simulink model "PIDController"  (R2019a)
settings: Solver=ode5  StartTime=0.0  StopTime=inf  FixedStep=0.01  RelTol=1e-3
settings Model: Creator=Admin  LastModifiedBy=Admin
settings DataIOCC: ReturnWorkspaceOutputs=off
settings DebuggingCC: ArithmeticOperatorsInVariantConditions=warning
settings SFSimCC: SimUseLocalCustomCode=off
settings RTWCC: RTWUseLocalCustomCode=off
settings CodeAppCC: StateflowObjectComments=on

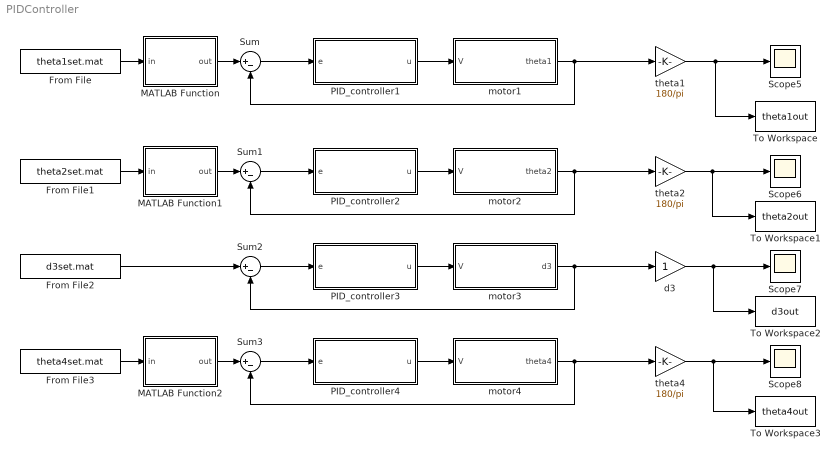
== system PIDController ==
  From File : FromFile  FileName=theta1set.mat
  From File1 : FromFile  FileName=theta2set.mat
  From File2 : FromFile  FileName=d3set.mat
  From File3 : FromFile  FileName=theta4set.mat
  MATLAB Function : MATLAB Function  TreatAsAtomicUnit=on
  MATLAB Function1 : MATLAB Function  TreatAsAtomicUnit=on
  MATLAB Function2 : MATLAB Function  TreatAsAtomicUnit=on
  PID_controller1 : Subsystem  mask{Kp=500, Ki=0, Kd=0}
  PID_controller2 : Subsystem  mask{Kp=500, Ki=0, Kd=0}
  PID_controller3 : Subsystem  mask{Kp=500, Ki=0, Kd=0}
  PID_controller4 : Subsystem  mask{Kp=500, Ki=0, Kd=0}
  Scope{5..8} (4 alike) : Scope
  Sum{,1..3} (4 alike) : Sum  Inputs=|+-
  To Workspace : ToWorkspace  VariableName=theta1out  SampleTime=-1
  To Workspace1 : ToWorkspace  VariableName=theta2out  SampleTime=-1
  To Workspace2 : ToWorkspace  VariableName=d3out  SampleTime=-1
  To Workspace3 : ToWorkspace  VariableName=theta4out  SampleTime=-1
  d3 : Gain
  motor1 : Subsystem  mask{Ki=0.1, Kb=0.1, L=0.5, R=2, Jeff=0.02, Beff=0.2, N=100}
  motor2 : Subsystem  mask{Ki=0.1, Kb=0.1, L=0.5, R=2, Jeff=0.02, Beff=0.2, N=100}
  motor3 : Subsystem  mask{Ki=0.1, Kb=0.1, L=0.5, R=2, Jeff=0.02, Beff=0.2, N=100}
  motor4 : Subsystem  mask{Ki=0.1, Kb=0.1, L=0.5, R=2, Jeff=0.02, Beff=0.2, N=100}
  theta1 : Gain  Gain=180/pi
  theta2 : Gain  Gain=180/pi
  theta4 : Gain  Gain=180/pi
  wires:
  Sum/1 -> PID_controller1/1(e)
  PID_controller1/1(u) -> motor1/1(V)
  Sum1/1 -> PID_controller2/1(e)
  PID_controller2/1(u) -> motor2/1(V)
  Sum2/1 -> PID_controller3/1(e)
  PID_controller3/1(u) -> motor3/1(V)
  Sum3/1 -> PID_controller4/1(e)
  PID_controller4/1(u) -> motor4/1(V)
  From File2/1 -> Sum2/1
  theta4/1 -> To Workspace3/1, Scope8/1
  theta1/1 -> To Workspace/1, Scope5/1
  theta2/1 -> To Workspace1/1, Scope6/1
  motor3/1(d3) -> d3/1, Sum2/2
  d3/1 -> To Workspace2/1, Scope7/1
  From File/1 -> MATLAB Function/1(in)
  From File1/1 -> MATLAB Function1/1(in)
  From File3/1 -> MATLAB Function2/1(in)
  motor4/1(theta4) -> theta4/1, Sum3/2
  motor2/1(theta2) -> theta2/1, Sum1/2
  motor1/1(theta1) -> theta1/1, Sum/2
  MATLAB Function/1(out) -> Sum/1
  MATLAB Function1/1(out) -> Sum1/1
  MATLAB Function2/1(out) -> Sum3/1

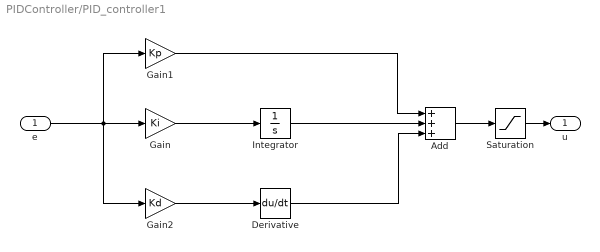
== system PIDController/PID_controller1 ==
  e : Inport
  Add : Sum  Inputs=+++
  Derivative : Derivative
  Gain : Gain  Gain=Ki
  Gain1 : Gain  Gain=Kp
  Gain2 : Gain  Gain=Kd
  Integrator : Integrator
  Saturation : Saturate  UpperLimit=300  LowerLimit=-300
  u : Outport
  wires:
  e/1 -> Gain2/1, Gain1/1, Gain/1
  Gain/1 -> Integrator/1
  Gain2/1 -> Derivative/1
  Gain1/1 -> Add/1
  Integrator/1 -> Add/2
  Derivative/1 -> Add/3
  Add/1 -> Saturation/1
  Saturation/1 -> u/1

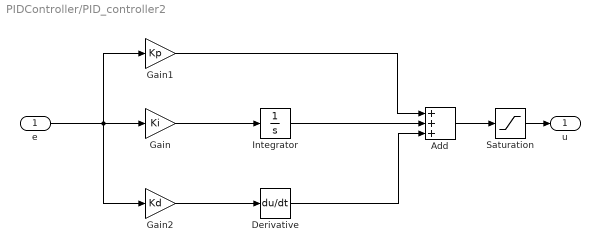
== system PIDController/PID_controller2 ==
  e : Inport
  Add : Sum  Inputs=+++
  Derivative : Derivative
  Gain : Gain  Gain=Ki
  Gain1 : Gain  Gain=Kp
  Gain2 : Gain  Gain=Kd
  Integrator : Integrator
  Saturation : Saturate  UpperLimit=300  LowerLimit=-300
  u : Outport
  wires:
  e/1 -> Gain2/1, Gain1/1, Gain/1
  Gain/1 -> Integrator/1
  Gain2/1 -> Derivative/1
  Gain1/1 -> Add/1
  Integrator/1 -> Add/2
  Derivative/1 -> Add/3
  Add/1 -> Saturation/1
  Saturation/1 -> u/1

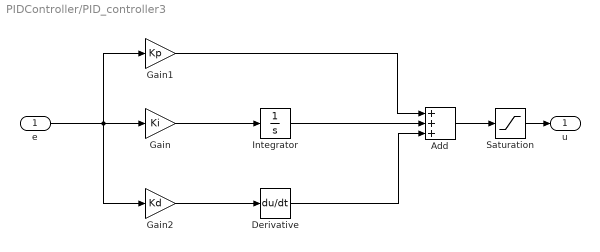
== system PIDController/PID_controller3 ==
  e : Inport
  Add : Sum  Inputs=+++
  Derivative : Derivative
  Gain : Gain  Gain=Ki
  Gain1 : Gain  Gain=Kp
  Gain2 : Gain  Gain=Kd
  Integrator : Integrator
  Saturation : Saturate  UpperLimit=300  LowerLimit=-300
  u : Outport
  wires:
  e/1 -> Gain2/1, Gain1/1, Gain/1
  Gain/1 -> Integrator/1
  Gain2/1 -> Derivative/1
  Gain1/1 -> Add/1
  Integrator/1 -> Add/2
  Derivative/1 -> Add/3
  Add/1 -> Saturation/1
  Saturation/1 -> u/1

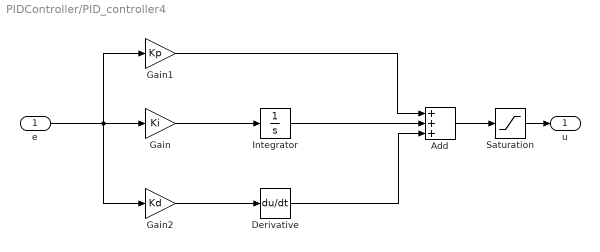
== system PIDController/PID_controller4 ==
  e : Inport
  Add : Sum  Inputs=+++
  Derivative : Derivative
  Gain : Gain  Gain=Ki
  Gain1 : Gain  Gain=Kp
  Gain2 : Gain  Gain=Kd
  Integrator : Integrator
  Saturation : Saturate  UpperLimit=300  LowerLimit=-300
  u : Outport
  wires:
  e/1 -> Gain2/1, Gain1/1, Gain/1
  Gain/1 -> Integrator/1
  Gain2/1 -> Derivative/1
  Gain1/1 -> Add/1
  Integrator/1 -> Add/2
  Derivative/1 -> Add/3
  Add/1 -> Saturation/1
  Saturation/1 -> u/1

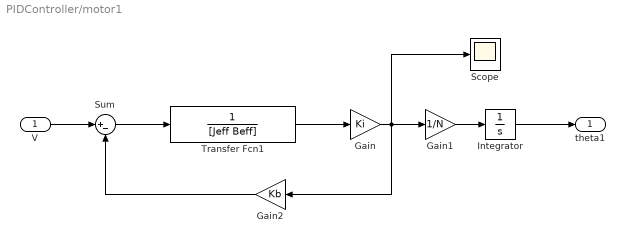
== system PIDController/motor1 ==
  V : Inport
  Gain : Gain  Gain=Ki
  Gain1 : Gain  Gain=1/N
  Gain2 : Gain  Gain=Kb
  Integrator : Integrator
  Scope : Scope
  Sum : Sum  Inputs=|+-
  Transfer Fcn1 : TransferFcn  Denominator=[Jeff Beff]
  theta1 : Outport
  wires:
  Transfer Fcn1/1 -> Gain/1
  Gain2/1 -> Sum/2
  V/1 -> Sum/1
  Sum/1 -> Transfer Fcn1/1
  Gain/1 -> Gain1/1, Gain2/1, Scope/1
  Gain1/1 -> Integrator/1
  Integrator/1 -> theta1/1

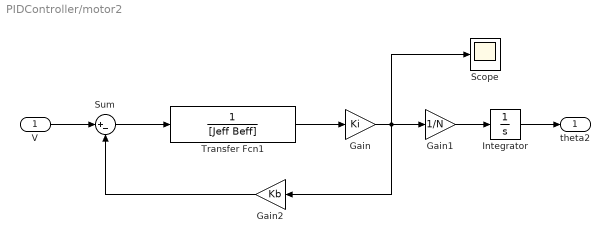
== system PIDController/motor2 ==
  V : Inport
  Gain : Gain  Gain=Ki
  Gain1 : Gain  Gain=1/N
  Gain2 : Gain  Gain=Kb
  Integrator : Integrator  InitialCondition=1.57
  Scope : Scope
  Sum : Sum  Inputs=|+-
  Transfer Fcn1 : TransferFcn  Denominator=[Jeff Beff]
  theta2 : Outport
  wires:
  Transfer Fcn1/1 -> Gain/1
  Gain1/1 -> Integrator/1
  Gain2/1 -> Sum/2
  V/1 -> Sum/1
  Sum/1 -> Transfer Fcn1/1
  Gain/1 -> Gain1/1, Gain2/1, Scope/1
  Integrator/1 -> theta2/1

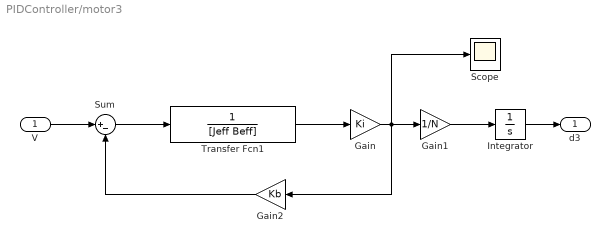
== system PIDController/motor3 ==
  V : Inport
  Gain : Gain  Gain=Ki
  Gain1 : Gain  Gain=1/N
  Gain2 : Gain  Gain=Kb
  Integrator : Integrator
  Scope : Scope
  Sum : Sum  Inputs=|+-
  Transfer Fcn1 : TransferFcn  Denominator=[Jeff Beff]
  d3 : Outport
  wires:
  Transfer Fcn1/1 -> Gain/1
  Gain1/1 -> Integrator/1
  Integrator/1 -> d3/1
  Gain2/1 -> Sum/2
  V/1 -> Sum/1
  Sum/1 -> Transfer Fcn1/1
  Gain/1 -> Gain1/1, Gain2/1, Scope/1

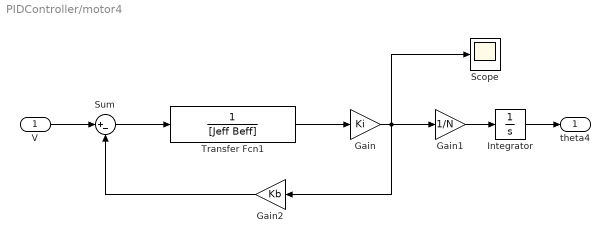
== system PIDController/motor4 ==
  V : Inport
  Gain : Gain  Gain=Ki
  Gain1 : Gain  Gain=1/N
  Gain2 : Gain  Gain=Kb
  Integrator : Integrator  InitialCondition=-1.57
  Scope : Scope
  Sum : Sum  Inputs=|+-
  Transfer Fcn1 : TransferFcn  Denominator=[Jeff Beff]
  theta4 : Outport
  wires:
  Transfer Fcn1/1 -> Gain/1
  Gain/1 -> Gain1/1, Gain2/1, Scope/1
  Gain1/1 -> Integrator/1
  Gain2/1 -> Sum/2
  V/1 -> Sum/1
  Sum/1 -> Transfer Fcn1/1
  Integrator/1 -> theta4/1

== matlab function PIDController/MATLAB Function1 ==
  settings: updateMethod=DISCRETE
  data: in input; out output
function out = HandleInput(in)

out = in
persistent pre
if isempty(pre)
    pre = 0;
end

while (out - pre > 1.5*pi)
    out = out - 2*pi;
end

while (out - pre < -1.5*pi)
    out = out + 2*pi;
end

== matlab function PIDController/MATLAB Function ==
  settings: updateMethod=DISCRETE
  data: in input; out output
function out = HandleInput(in)

out = in
persistent pre
if isempty(pre)
    pre = 0;
end

while (out - pre > 1.5*pi)
    out = out - 2*pi;
end

while (out - pre < -1.5*pi)
    out = out + 2*pi;
end

== matlab function PIDController/MATLAB Function2 ==
  settings: updateMethod=DISCRETE
  data: in input; out output
function out = HandleInput(in)

out = in;
persistent pre
if isempty(pre)
    pre = 0;
end

while (out - pre > 1.5*pi)
    out = out - 2*pi;
end

while (out - pre < -1.5*pi)
    out = out + 2*pi;
end
